simulink model "MMMS_v1_dynamics"  (R2024a)
settings: Solver=VariableStepAuto  StartTime=0.0  StopTime=120  FixedStep=0.001  RelTol=1e-3
InitFcn:
  | %rho_0t=[0.29;0.29;0.29]; %m
  | %V_0t=[-0.001;-0.001;0];%[-0.0005;-0.0005;0];
  | %w_t=[0;0;-0.002];
  | 
  | 
  | %rho_0t=[0.3;0.3;0.2]; %m
  | %V_0t=[-0.001;-0.001;0];%[-0.0005;-0.0005;0];
  | %w_t=[0;0;-0.001];
values from neighbouring files (symbols this model uses):
  Dt = 0.1    [main_EKF.m]
  g_cm = zeros(4,4,n)    [Initiate_KUKA_inv.m]    (also in Main_MMMS.m; test_KUKA_elements.m)
  g_It00 = [eye(3) rho_It;0 0 0 1]    [main_EKF.m]
  iota0 = eye(6,6)    [Initiate_KUKA_inv.m]    (also in Main_MMMS.m; test_KUKA_elements.m)
  K_d = 10*[1.3*eye(3) zeros(3);zeros(3) 0.8*eye(3)]    [Initiate_FQ.m]    (also in Initiate_KUKA_inv.m = 5*[0.7*eye(3) zeros(3);zeros(3) 0.5*eye(3)]; MMMS_Initiate_FQ.m; Main_MMMS.m = 5*[0.7*eye(3) zeros(3);zeros(3) 0.5*eye(3)]; test_KUKA_elements.m = 50*[0.7*eye(3) zeros(3);zeros(3) 0.5*eye(3)])
  K_i = 5*[0.1*eye(3) zeros(3);zeros(3) 0.01*eye(3)]    [Initiate_FQ.m]    (also in Initiate_KUKA_inv.m = 5*[0.01*eye(3) zeros(3);zeros(3) 0.001*eye(3)]; MMMS_Initiate_FQ.m; Main_MMMS.m = 5*[0.01*eye(3) zeros(3);zeros(3) 0.001*eye(3)]; test_KUKA_elements.m = 50*[0.01*eye(3) zeros(3);zeros(3) 0.001*eye(3)])
  K_p = 100*[0.1 0 0 0 0 0;0 0.1 0 0 0 0; 0 0 0.1 0 0 0; 0 0 0 0.01 0 0 ... (first row only)    [Initiate_FQ.m]    (also in Initiate_KUKA_inv.m = 5*[0.1 0 0 0 0 0;0 0.1 0 0 0 0; 0 0 0.1 0 0 0; 0 0 0 0.01 0 ; MMMS_Initiate_FQ.m; Main_MMMS.m = 5*[0.1 0 0 0 0 0;0 0.1 0 0 0 0; 0 0 0.1 0 0 0; 0 0 0 0.01 0 ; test_KUKA_elements.m = 50*[0.1 0 0 0 0 0;0 0.1 0 0 0 0; 0 0 0.1 0 0 0; 0 0 0 0.01 0)
  K_w = 200*eye(7)    [Initiate_FQ.m]    (also in MMMS_Initiate_FQ.m)
  K_wd = 2*eye(7)    [Initiate_FQ.m]    (also in MMMS_Initiate_FQ.m)
  m = randn(s,total_time_steps,6)*chol(R)    [main_EKF.m]
  M0 = M_temp.M0.data(:,:,1)    [Initiate_FQ.m]    (also in MMMS_Initiate_FQ.m; test_KUKA_elements.m)
  m0 = robot.Bodies{1,n+1}.Mass    [Initiate_KUKA_inv.m]    (also in Main_MMMS.m; test_KUKA_elements.m)
  m0_frak = diag_M(1:6,1:6)    [Initiate_KUKA_inv.m]    (also in Main_MMMS.m; make_uncertain.m = diag_M_unc(1:6,1:6); test_KUKA_elements.m)
  M0m = M_temp.M0m.data(:,:,1)    [Initiate_FQ.m]    (also in MMMS_Initiate_FQ.m; test_KUKA_elements.m)
  m_diag = diag_M(7:end,7:end)    [Initiate_KUKA_inv.m]    (also in Main_MMMS.m; make_uncertain.m = diag_M_unc(7:end,7:end); test_KUKA_elements.m)
  M_t = (((Adjoint(g_It))'\M_t_body)/(Adjoint(g_It)))    [Initiate_FQ.m]    (also in Initiate_KUKA_inv.m = [eye(3)*mt zeros(3); zeros(3) eye(3)*80]; MMMS_Initiate_FQ.m; Main_MMMS.m = [eye(3)*mt zeros(3); zeros(3) eye(3)*80]; test_KUKA_elements.m = [eye(3)*mt zeros(3); zeros(3) eye(3)*80])
  M_t_body = [eye(3)*mt zeros(3); zeros(3) eye(3)*0.416667]    [Initiate_FQ.m]    (also in MMMS_Initiate_FQ.m)
  mm = zeros(1,n)    [Initiate_KUKA_inv.m]    (also in Main_MMMS.m; test_KUKA_elements.m)
  mu = P0    [Initiate_FQ.m]    (also in Initiate_KUKA_inv.m = zeros(6,1); MMMS_Initiate_FQ.m; Main_MMMS.m = zeros(6,1); make_uncertain.m = P0_unc)
  mu_t = inv((Adjoint(g_It))')*M_t_body*[V_It;w_t]    [Initiate_FQ.m]    (also in Initiate_KUKA_inv.m = M_t*[V_0t;w_t]; MMMS_Initiate_FQ.m; Main_MMMS.m = M_t*[V_0t;w_t]; make_uncertain.m = inv((Adjoint(g_It))')*M_t_body_unc*[V_It;w_t])
  noise_st = 0.000005    (= 5e-06)    [main_EKF.m]
  q_dot_m = [0;0;0;0;0;0;0]    [Initiate_FQ.m]    (also in Initiate_KUKA_inv.m; MMMS_Initiate_FQ.m; Main_MMMS.m; test_KUKA_elements.m = [0])
  q_m = [0.2;1.2;0.3;2.5;0.5;1.5;0.6]    [Initiate_FQ.m]    (also in Initiate_KUKA_inv.m = [0;0;0;0;0;0;0]; MMMS_Initiate_FQ.m = [0.2;0.2;0.3;0.5;0.5;0.5;0.6]; Main_MMMS.m = [0;0;0;0;0;0;0]; test_KUKA_elements.m = [0.2;1.2;0.3;1.8;0.5;1.3;0.6])
  rho_It = [-0.3;-0.3;-0.1]    [Initiate_FQ.m]    (also in MMMS_Initiate_FQ.m = [0;0;1.7])
  s = RandStream.create('mrg32k3a','NumStreams',1)    [main_EKF.m]
  sc_size = 1    [Initiate_KUKA_inv.m]    (also in Main_MMMS.m; test_KUKA_elements.m)
  V_It = [0.01;0.01;0]    [Initiate_FQ.m]    (also in MMMS_Initiate_FQ.m = [0.001;0.001;0])
  Xi_m_matrix = zeros(6*n,n)    [Initiate_KUKA_inv.m]    (also in Main_MMMS.m)
undefined symbols (not defined in the file or in its folder): g_cm0, I0, Im, Mm, X, Xi_m, Y, Z
libraries: nesl_utility x314, sm_lib x231, robotcorelib x30, simulink x12
(part 1 of 13)
settings Model: Creator=Bmmog  LastModifiedBy=Bmmog
settings SolverCC: ZeroCrossAlgorithm=Adaptive
settings DataIOCC: ReturnWorkspaceOutputsName=tp1ae71780_9f9b_41fc_80d6_93119145c185
settings DebuggingCC: UnconnectedInputMsg=warning  UnconnectedOutputMsg=warning  UnconnectedLineMsg=warning
settings ModelReferenceCC: EnableRefExpFcnMdlSchedulingChecks=on
settings RTWCC: GPUComputeCapability=3.5  DLArmComputeVersion=19.05
settings ExplorerConfigSet: InternalSimMechanicsExplorerSettings="<ExplorerConfiguration><canonicalview>default</canonicalview><AnimationSetting><BasePlaybackSpeed>1.0</BasePlaybackSpeed><PlaybackSpeedFactor>8.0</PlaybackSpeedFactor></AnimationSetting><TilePanel><TileInfo><Tiles Columns=\"1\" Count=\"1\" Rows=\"1\"><Column Weight=\"1\"/><Row Weight=\"1\"/><Tile Height=\"1\" Width=\"1\" X=\"0\" Y=\"0\"/></Tiles></TileInfo><SceneInfo><SceneViewer><BGColor><R>1</R><G>1</G><B>1</B></BGColor><Camera><DoPerspective>off</DoPerspective><Position><X>14.9326991217614395</X><Y>-1.09548928723552041</Y><Z>10.2239075521242828</Z></Position><Center><X>11.9633929326695281</X><Y>-0.827691225044008383</Y><Z>8.31444606315609391</Z></Center><Up><X>-0.521882593040954079</X><Y>0.171482170510200094</Y><Z>0.835603030318799456</Z></Up><ViewLimDist>1</ViewLimDist><YLim>2.32554507561611068</YLim><XLim>3.37013417515515057</XLim></Camera></SceneViewer></SceneInfo></TilePanel><MechEditorPanel><Cameras/><GfxPanelCameraMap/><VideoCreator><PlaybackSpeedRatio>1.0</PlaybackSpeedRatio><FrameRate>30</FrameRate><VideoFormat>Motion JPEG AVI</VideoFormat><FrameSize>auto</FrameSize></VideoCreator></MechEditorPanel></ExplorerConfiguration>"

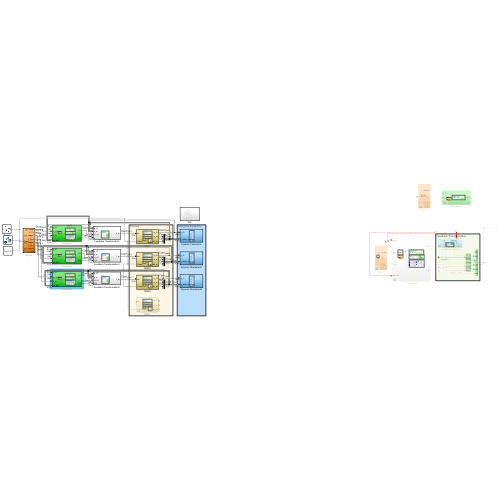
[thumbnail: Simulink's stored preview of the top-level diagram]
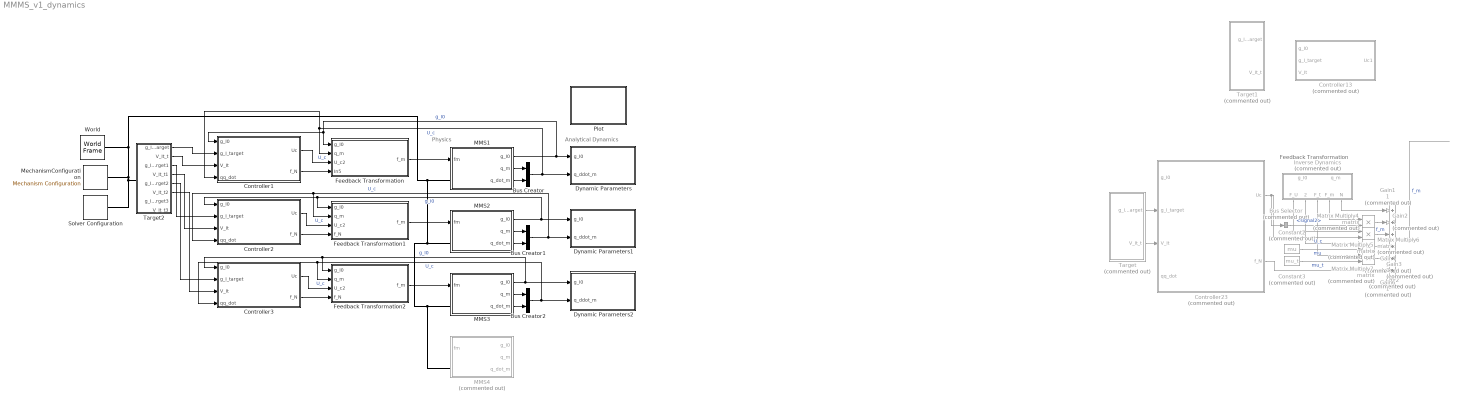
== system MMMS_v1_dynamics ==
  note: Analytical Dynamics
  note: Physics
  note: Feedback Transformation
  Add2 : Sum  Commented=on  Inputs=++++++
  Bus Creator : BusCreator  Inputs=2
  Bus Creator1 : BusCreator  Inputs=2
  Bus Creator2 : BusCreator  Inputs=2
  Bus Selector : BusSelector  Commented=on  OutputSignals=signal2
  Constant2 : Constant  Commented=on  Value=mu
  Constant3 : Constant  Commented=on  Value=mu_t
  Controller1 : Subsystem
  Controller13 : Subsystem  Commented=on
  Controller2 : Subsystem
  Controller23 : Subsystem  Commented=on
  Controller3 : Subsystem
  Dynamic Parameters : Subsystem
  Dynamic Parameters1 : Subsystem
  Dynamic Parameters2 : Subsystem
  Feedback Transformation : Subsystem
  Feedback Transformation1 : Subsystem
  Feedback Transformation2 : Subsystem
  Gain{1..4,6} (5 alike) : Gain  Commented=on
  Inverse Dynamics : Subsystem  Commented=on
  MMS1 : Subsystem
  MMS2 : Subsystem
  MMS3 : Subsystem
  MMS4 : Subsystem  Commented=on
  Matrix Multiply{4..7} (4 alike) : Product  Commented=on  Multiplication=Matrix(*)
  MechanismConfiguration : sm_lib/Utilities/Mechanism Configuration  UniformGravity=Constant  GravityVector=[0 0 0]  GravityVectorUnits=m/s^2  LinearizationDelta=0.001  JointModeTransitionNonlinearIterations=2
  Plot : Subsystem
  Solver Configuration : nesl_utility/Solver Configuration  PhysicalDomain=network_engine_domain  SubClassName=solver  LeftPortType=input  RightPortType=generic  Tones=[]  Harmonics=[]  SimulateNoise=off  Profile=off  UseLocalSampling=off  EnableSwitchedLinearOptims=on  FrequencyDomain=off  UseCCode=off  RelTol=0.001  AbsTol=0.001  MinStep=1e-09  ToWorkspace=off  RevertToSquareIcSolve=off  NumHomotopyIterations=100  PhasorMode=off  PhasorModeNumHarmonics=1  ConsistencySolver=NEWTON_FTOL  IndexReductionMethod=DerivativeReplacement  DoDC=off  ResidualTolerance=1e-9  ConsistencyTolSource=GLOBAL  ConsistencyAbsTol=0.001  ConsistencyRelTol=0.001  ConsistencyTolFactor=0.001  UseLocalSolver=off  LocalSolverChoice=NE_BACKWARD_EULER_ADVANCER  ResolveIndetEquations=on  FunctionEvalNumThread=1  LocalSolverSampleTime=0.001  DoFixedCost=off  MaxNonlinIter=3  MaxModeIter=2  ComputeImpulses=off  ImpulseIterations=2  LinearAlgebra=Full  LinearAlgebraNumThread=0  EquationFormulation=NE_TIME_EF  DelaysMemoryBudget=1024  AutomaticFiltering=off  FilteringTimeConstant=0.001  PartitionStorageMethod=AS_NEEDED  PartitionMemoryBudget=1024  PartitionMethod=ROBUST  MultibodyUseLocalSolver=off  MultibodyLocalSolverChoice=ODE1  MultibodyLocalSolverSampleTime=0.001
  Target : Subsystem  Commented=on
  Target1 : Subsystem  Commented=on
  Target2 : Subsystem
  World : sm_lib/Frames and Transforms/World Frame
  wires:
  MMS1/2(q_m) -> Bus Creator/1
  MMS1/3(q_dot_m) -> Bus Creator/2
  Gain3/1 -> Add2/5
  Constant3/1 -> Matrix Multiply7/2  "mu_t"
  Controller23/2(f_N) -> Gain6/1
  Gain4/1 -> Add2/4
  Inverse Dynamics/1(F_U) -> Matrix Multiply5/1
  Inverse Dynamics/5(N) -> Gain1/1
  Gain6/1 -> Add2/6
  Matrix Multiply6/1 -> Gain4/1
  Matrix Multiply7/1 -> Gain3/1
  Gain2/1 -> Add2/2
  Inverse Dynamics/2(F_mu) -> Matrix Multiply6/1
  Target/1(g_I_target) -> Controller23/2(g_I_target)
  Inverse Dynamics/4(F_m) -> Matrix Multiply4/1
  Add2/1 -> ?  "f_m"
  Gain1/1 -> Add2/1
  Constant2/1 -> Matrix Multiply6/2  "mu"
  Controller23/1(Uc) -> Matrix Multiply5/2, Bus Selector/1  "U_c"
  Inverse Dynamics/3(F_t) -> Matrix Multiply7/1
  Matrix Multiply5/1 -> Add2/3  "f_m"
  ? -> Controller23/4(qq_dot)
  Matrix Multiply4/1 -> Gain2/1
  ? -> Inverse Dynamics/2("q_m ")
  ? -> Controller23/1(g_I0)  "g_I0"
  Target/2(V_It_t) -> Controller23/3(V_It)
  Bus Selector/1 -> Matrix Multiply4/2  "<signal2>"
  Bus Creator/1 -> Feedback Transformation/2(q_m), Controller1/4(qq_dot), Dynamic Parameters/2(q_ddot_m)  "U_c"
  Target2/1(g_I_target) -> Controller1/2(g_I_target)
  Target2/2(V_It_t) -> Controller1/3(V_It)
  MMS1/1(g_I0) -> Controller1/1(g_I0), Feedback Transformation/1(g_I0), Dynamic Parameters/1(g_I0)  "g_I0"
  Controller1/1(Uc) -> Feedback Transformation/3(U_c2)  "U_c"
  Controller1/2(f_N) -> Feedback Transformation/4(In5)
  Feedback Transformation/1(f_m) -> MMS1/1(fm)
  MMS2/2(q_m) -> Bus Creator1/1
  MMS2/3(q_dot_m) -> Bus Creator1/2
  MMS2/1(g_I0) -> Feedback Transformation1/1(g_I0), Controller2/1(g_I0), Dynamic Parameters1/1(g_I0)  "g_I0"
  Bus Creator1/1 -> Feedback Transformation1/2(q_m), Controller2/4(qq_dot), Dynamic Parameters1/2(q_ddot_m)  "U_c"
  Controller2/1(Uc) -> Feedback Transformation1/3(U_c2)  "U_c"
  Controller2/2(f_N) -> Feedback Transformation1/4(f_N)
  Target2/3(g_I_target1) -> Controller2/2(g_I_target)
  Target2/4(V_It_t1) -> Controller2/3(V_It)
  Feedback Transformation1/1(f_m) -> MMS2/1(fm)
  MMS3/1(g_I0) -> Feedback Transformation2/1(g_I0), Controller3/1(g_I0), Dynamic Parameters2/1(g_I0)  "g_I0"
  MMS3/2(q_m) -> Bus Creator2/1
  MMS3/3(q_dot_m) -> Bus Creator2/2
  Bus Creator2/1 -> Feedback Transformation2/2(q_m), Controller3/4(qq_dot), Dynamic Parameters2/2(q_ddot_m)  "U_c"
  Controller3/2(f_N) -> Feedback Transformation2/4(f_N)
  Controller3/1(Uc) -> Feedback Transformation2/3(U_c2)  "U_c"
  Target2/5(g_I_target2) -> Controller3/2(g_I_target)
  Target2/6(V_It_t2) -> Controller3/3(V_It)
  Feedback Transformation2/1(f_m) -> MMS3/1(fm)
  connections:
  MechanismConfiguration/RConn1 -- Target2/LConn1 -- Solver Configuration/RConn1 -- MMS4/LConn1 -- MMS3/LConn1 -- MMS2/LConn1 -- MMS1/LConn1 -- World/RConn1

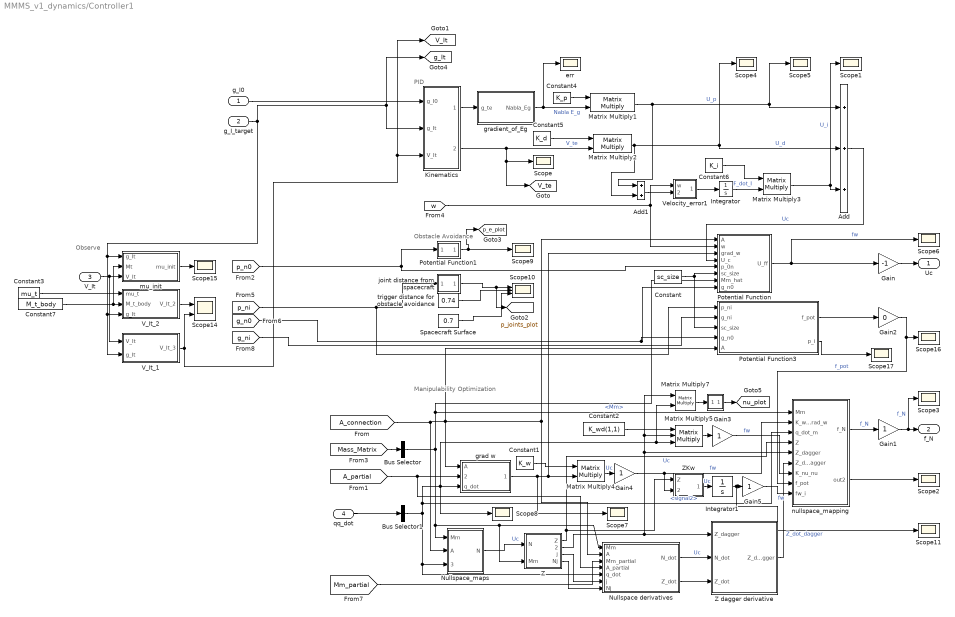
== system MMMS_v1_dynamics/Controller1 ==
  note: PID
  note: Manipulability Optimization
  note: Obstacle Avoidance
  note: Observe
  g_I0 : Inport
  g_I_target : Inport  Port=2
  V_It : Inport  Port=3
  qq_dot : Inport  Port=4
  " " : MATLAB Function  TreatAsAtomicUnit=on
  Add : Sum  Inputs=+++
  Add1 : Sum
  Bus Selector : BusSelector  OutputSignals=Mm
  Bus Selector1 : BusSelector  OutputSignals=signal2
  Constant : Constant  Value=sc_size
  Constant1 : Constant  Value=K_w
  Constant2 : Constant  Value=K_wd(1,1)
  Constant3 : Constant  Value=mu_t
  Constant4 : Constant  Value=K_p
  Constant5 : Constant  Value=K_d
  Constant6 : Constant  Value=K_i
  Constant7 : Constant  Value=M_t_body
  Gain : Gain  Gain=-1
  Gain{1,3..5} (4 alike) : Gain
  Gain2 : Gain  Gain=0
  Integrator : Integrator
  Integrator1 : Integrator
  Kinematics : Subsystem
  Matrix Multiply{1..4,7} (5 alike) : Product  Multiplication=Matrix(*)
  Matrix Multiply5 : Product  Inputs=3  Multiplication=Matrix(*)
  Nullspace derivatives : MATLAB Function  TreatAsAtomicUnit=on
  Nullspace_maps : MATLAB Function  TreatAsAtomicUnit=on
  Potential Function : MATLAB Function  TreatAsAtomicUnit=on
  Potential Function1 : MATLAB Function  TreatAsAtomicUnit=on
  Potential Function3 : MATLAB Function  TreatAsAtomicUnit=on
  Scope{,1..9,11,15..17} (14 alike) : Scope
  Scope10 : Scope  NumInputPorts=3
  Scope14 : Scope  NumInputPorts=2
  Spacecraft Surface : Constant  Value=0.7
  V_It_1 : MATLAB Function  TreatAsAtomicUnit=on
  V_It_2 : MATLAB Function  TreatAsAtomicUnit=on
  Velocity_error1 : MATLAB Function  TreatAsAtomicUnit=on
  Z : MATLAB Function  TreatAsAtomicUnit=on
  Z dagger derivative : MATLAB Function  TreatAsAtomicUnit=on
  ZKw : MATLAB Function  TreatAsAtomicUnit=on
  err : Scope
  grad w : MATLAB Function  TreatAsAtomicUnit=on
  gradient_of_Eg : MATLAB Function  TreatAsAtomicUnit=on
  joint distance from spacecraft : MATLAB Function  TreatAsAtomicUnit=on
  mu_init : MATLAB Function  TreatAsAtomicUnit=on
  nullspace_mapping : MATLAB Function  TreatAsAtomicUnit=on
  trigger distance for obstacle avoidance : Constant  Value=0.74
  Uc : Outport
  f_N : Outport  Port=2
  tag scope: V_It=global, V_te=global, g_It=global, nu_plot=global, p_e_plot=global, p_joints_plot=global
  wires:
  [A_connection] -> Potential Function3/5(A), Potential Function/1(A), Nullspace derivatives/2(A), grad w/1(A), Nullspace_maps/2(A)
  [A_partial] -> grad w/2(A_partial), Nullspace derivatives/4(A_partial)
  qq_dot/1 -> Bus Selector1/1
  [Mass_Matrix] -> Bus Selector/1
  Bus Selector/1 -> Nullspace_maps/1(Mm), Z/2(Mm), Nullspace derivatives/1(Mm), Potential Function/7(Mm_hat), nullspace_mapping/1(Mm)  "<Mm>"
  Gain/1 -> Uc/1
  g_I0/1 -> Kinematics/1(g_I0)
  Add/1 -> Potential Function/4(U_c)  "Uc"
  Kinematics/1(g_te1) -> gradient_of_Eg/1(g_te)
  Add1/1 -> Velocity_error1/2(in)
  Matrix Multiply2/1 -> Scope4/1, Add/2, Add1/2  "U_d"
  gradient_of_Eg/1(Nabla_Eg) -> err/1, Matrix Multiply1/2  "Nabla E_g"
  Constant4/1 -> Matrix Multiply1/1
  Kinematics/2(V_te) -> [V_te], Scope/1, Matrix Multiply2/2  "V_te"
  Constant6/1 -> Matrix Multiply3/1
  Integrator/1 -> Matrix Multiply3/2  "F_dot_I"
  Matrix Multiply1/1 -> Scope5/1, Add/1, Add1/1  "U_p"
  Constant5/1 -> Matrix Multiply2/1
  Bus Selector1/1 -> nullspace_mapping/3(q_dot_m), Scope8/1, grad w/3(q_dot), Matrix Multiply7/2, Matrix Multiply5/3, Nullspace derivatives/5(q_dot), Nullspace_maps/3(q_dot_m)  "<signal2>"
  Gain1/1 -> f_N/1, Scope3/1  "f_N"
  Constant1/1 -> Matrix Multiply4/1
  grad w/1(grad_w) -> Scope7/1, Potential Function/3(grad_w), Matrix Multiply4/2
  Matrix Multiply5/1 -> Gain3/1
  Constant2/1 -> Matrix Multiply5/1
  Matrix Multiply4/1 -> Gain4/1  "Uc"
  Matrix Multiply3/1 -> Scope1/1, Add/3  "U_i"
  nullspace_mapping/1(f_N) -> Gain1/1  "f_N"
  [w] -> Potential Function/2(w), Velocity_error1/1(w)
  Potential Function/1(U_ff) -> Gain/1, Scope6/1  "fw"
  Velocity_error1/1(out) -> Integrator/1
  [p_n0] -> Potential Function1/1(p_0n), Potential Function/5(p_0n)
  Potential Function1/1(w_p) -> Scope9/1, [p_e_plot]
  [p_ni] -> joint distance from spacecraft/1(p_joints), Potential Function3/1(p_ni)
  joint distance from spacecraft/1(pnorm) -> [p_joints_plot], Scope10/1
  [g_n0] -> Potential Function3/4(g_n0), Potential Function/8(g_n0)
  Potential Function3/1(f_pot) -> Gain2/1
  Constant/1 -> Potential Function3/3(sc_size), Potential Function/6(sc_size)
  trigger distance for obstacle avoidance/1 -> Scope10/2
  Gain3/1 -> nullspace_mapping/7(K_nu_nu)  "fw"
  Nullspace derivatives/1(N_dot) -> Z dagger derivative/2(N_dot)  "Uc"
  Nullspace derivatives/2(Z_dot) -> Z dagger derivative/3(Z_dot)
  Z dagger derivative/1(Z_dot_dagger) -> nullspace_mapping/6(Z_dot_dagger)  "Z_dot_dagger"
  Nullspace_maps/1(N) -> Z/1(N)  "Uc"
  [Mm_partial] -> Nullspace derivatives/3(Mm_partial)
  Z/1(Z) -> ZKw/1(Z), nullspace_mapping/4(Z)  "Uc"
  Gain4/1 -> ZKw/2(K_w_grad_w), nullspace_mapping/2(K_w_grad_w)  "fw"
  nullspace_mapping/2(out2) -> Scope2/1
  Z/2(Z_dagger) -> Z dagger derivative/1(Z_dagger), nullspace_mapping/5(Z_dagger), Matrix Multiply7/1, Matrix Multiply5/2
  ZKw/1(out) -> Integrator1/1  "Uc"
  Integrator1/1 -> Scope11/1, Gain5/1
  Gain5/1 -> nullspace_mapping/9(fw_i)  "fw"
  V_It/1 -> V_It_1/1(V_It), mu_init/3(V_It)
  Constant3/1 -> V_It_2/1(mu_t)
  mu_init/1(mu_init) -> Scope15/1
  Constant7/1 -> mu_init/2(Mt), V_It_2/2(M_t_body)
  Gain2/1 -> Scope16/1, nullspace_mapping/8(f_pot)  "f_pot"
  Z/3(j) -> Nullspace derivatives/6(j)
  Z/4(Nj) -> Nullspace derivatives/7(Nj)
  V_It_2/1(V_It_2) -> Scope14/1
  V_It_1/1(V_It_3) -> Scope14/2, Kinematics/3(V_It), [V_It]
  Spacecraft Surface/1 -> Scope10/3
  [g_ni] -> Potential Function3/2(g_ni)
  Potential Function3/2(p_i) -> Scope17/1
  g_I_target/1 -> Kinematics/2(g_It), [g_It], V_It_1/2(g_It), V_It_2/3(g_It), mu_init/1(g_It)
  " "/1(normA) -> [nu_plot]
  Matrix Multiply7/1 -> " "/1(A)

== system MMMS_v1_dynamics/Controller13 ==
  note: PID
  note: Observe
  g_I0 : Inport
  g_I_target : Inport  Port=2
  V_It : Inport  Port=3
  Add : Sum  Inputs=+++
  Add1 : Sum
  Constant3 : Constant  Value=mu_t
  Constant4 : Constant  Value=K_p
  Constant5 : Constant  Value=K_d
  Constant6 : Constant  Value=K_i
  Constant7 : Constant  Value=M_t_body
  From4 : From  Commented=on  GotoTag=w
  Gain1 : Gain  Gain=-1
  Integrator : Integrator
  Kinematics : Subsystem
  Matrix Multiply1 : Product  Multiplication=Matrix(*)
  Matrix Multiply2 : Product  Multiplication=Matrix(*)
  Matrix Multiply3 : Product  Multiplication=Matrix(*)
  Scope : Scope
  Scope1 : Scope  NumInputPorts=3
  Scope14 : Scope  NumInputPorts=2
  Scope15 : Scope
  V_It_1 : MATLAB Function  TreatAsAtomicUnit=on
  V_It_2 : MATLAB Function  TreatAsAtomicUnit=on
  Velocity_error1 : MATLAB Function  Commented=on  TreatAsAtomicUnit=on
  err : Scope
  gradient_of_Eg : MATLAB Function  TreatAsAtomicUnit=on
  mu_init : MATLAB Function  TreatAsAtomicUnit=on
  Uc1 : Outport
  tag scope: V_It=global, V_te=global, g_It=global
  wires:
  g_I0/1 -> Kinematics/1(g_I0)
  Kinematics/1(g_te1) -> gradient_of_Eg/1(g_te)
  Matrix Multiply2/1 -> Add/2, Scope1/2, Add1/2  "U_d"
  gradient_of_Eg/1(Nabla_Eg) -> err/1, Matrix Multiply1/2  "Nabla E_g"
  Constant4/1 -> Matrix Multiply1/1
  Kinematics/2(V_te) -> [V_te], Scope/1, Matrix Multiply2/2  "V_te"
  Constant6/1 -> Matrix Multiply3/1
  Integrator/1 -> Matrix Multiply3/2  "F_dot_I"
  Matrix Multiply1/1 -> Scope1/1, Add/1, Add1/1  "U_p"
  Constant5/1 -> Matrix Multiply2/1
  Matrix Multiply3/1 -> Add/3, Scope1/3  "U_i"
  From4/1 -> Velocity_error1/1(w)
  Add1/1 -> Integrator/1
  V_It/1 -> V_It_1/1(V_It), mu_init/3(V_It)
  Constant3/1 -> V_It_2/1(mu_t)
  mu_init/1(mu_init) -> Scope15/1
  Constant7/1 -> mu_init/2(Mt), V_It_2/2(M_t_body)
  V_It_2/1(V_It_2) -> Scope14/1
  V_It_1/1(V_It_3) -> Scope14/2, Kinematics/3(V_It), [V_It]
  g_I_target/1 -> [g_It], Kinematics/2(g_It), V_It_1/2(g_It), V_It_2/3(g_It), mu_init/1(g_It)
  Add/1 -> Gain1/1  "Uc"
  Gain1/1 -> Uc1/1

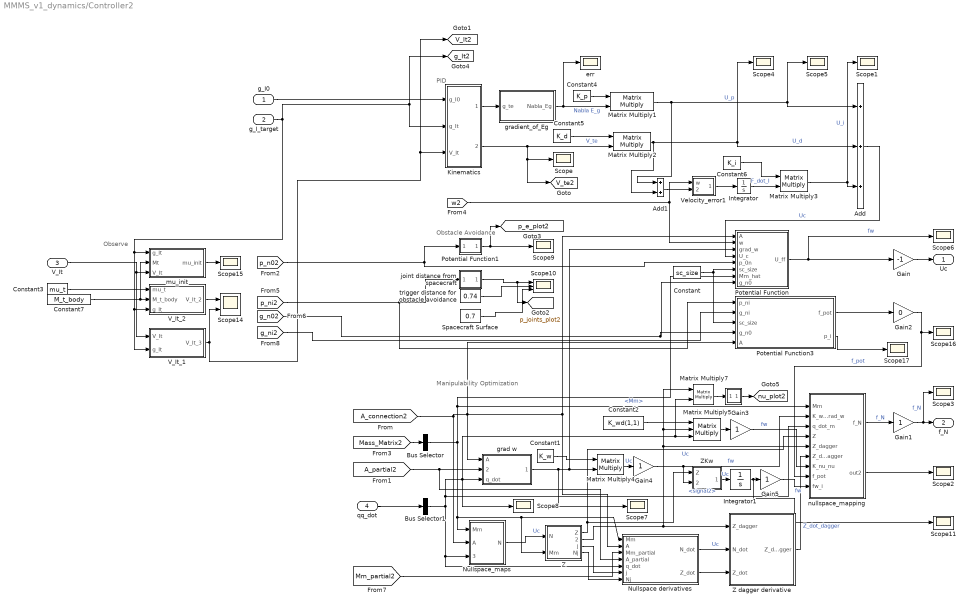
== system MMMS_v1_dynamics/Controller2 ==
  note: Observe
  note: Obstacle Avoidance
  note: Manipulability Optimization
  note: PID
  g_I0 : Inport
  g_I_target : Inport  Port=2
  V_It : Inport  Port=3
  qq_dot : Inport  Port=4
  " " : MATLAB Function  TreatAsAtomicUnit=on
  Add : Sum  Inputs=+++
  Add1 : Sum
  Bus Selector : BusSelector  OutputSignals=Mm
  Bus Selector1 : BusSelector  OutputSignals=signal2
  Constant : Constant  Value=sc_size
  Constant1 : Constant  Value=K_w
  Constant2 : Constant  Value=K_wd(1,1)
  Constant3 : Constant  Value=mu_t
  Constant4 : Constant  Value=K_p
  Constant5 : Constant  Value=K_d
  Constant6 : Constant  Value=K_i
  Constant7 : Constant  Value=M_t_body
  Gain : Gain  Gain=-1
  Gain{1,3..5} (4 alike) : Gain
  Gain2 : Gain  Gain=0
  Integrator : Integrator
  Integrator1 : Integrator
  Kinematics : Subsystem
  Matrix Multiply{1..4,7} (5 alike) : Product  Multiplication=Matrix(*)
  Matrix Multiply5 : Product  Inputs=3  Multiplication=Matrix(*)
  Nullspace derivatives : MATLAB Function  TreatAsAtomicUnit=on
  Nullspace_maps : MATLAB Function  TreatAsAtomicUnit=on
  Potential Function : MATLAB Function  TreatAsAtomicUnit=on
  Potential Function1 : MATLAB Function  TreatAsAtomicUnit=on
  Potential Function3 : MATLAB Function  TreatAsAtomicUnit=on
  Scope{,1..9,11,15..17} (14 alike) : Scope
  Scope10 : Scope  NumInputPorts=3
  Scope14 : Scope  NumInputPorts=2
  Spacecraft Surface : Constant  Value=0.7
  V_It_1 : MATLAB Function  TreatAsAtomicUnit=on
  V_It_2 : MATLAB Function  TreatAsAtomicUnit=on
  Velocity_error1 : MATLAB Function  TreatAsAtomicUnit=on
  Z : MATLAB Function  TreatAsAtomicUnit=on
  Z dagger derivative : MATLAB Function  TreatAsAtomicUnit=on
  ZKw : MATLAB Function  TreatAsAtomicUnit=on
  err : Scope
  grad w : MATLAB Function  TreatAsAtomicUnit=on
  gradient_of_Eg : MATLAB Function  TreatAsAtomicUnit=on
  joint distance from spacecraft : MATLAB Function  TreatAsAtomicUnit=on
  mu_init : MATLAB Function  TreatAsAtomicUnit=on
  nullspace_mapping : MATLAB Function  TreatAsAtomicUnit=on
  trigger distance for obstacle avoidance : Constant  Value=0.74
  Uc : Outport
  f_N : Outport  Port=2
  tag scope: V_It2=global, V_te2=global, g_It2=global, nu_plot2=global, p_e_plot2=global, p_joints_plot2=global
  wires:
  Matrix Multiply7/1 -> " "/1(A)
  " "/1(normA) -> [nu_plot2]
  g_I_target/1 -> mu_init/1(g_It), V_It_2/3(g_It), V_It_1/2(g_It), [g_It2], Kinematics/2(g_It)
  Potential Function3/2(p_i) -> Scope17/1
  [g_ni2] -> Potential Function3/2(g_ni)
  Spacecraft Surface/1 -> Scope10/3
  V_It_1/1(V_It_3) -> [V_It2], Kinematics/3(V_It), Scope14/2
  V_It_2/1(V_It_2) -> Scope14/1
  Z/4(Nj) -> Nullspace derivatives/7(Nj)
  Z/3(j) -> Nullspace derivatives/6(j)
  Gain2/1 -> nullspace_mapping/8(f_pot), Scope16/1  "f_pot"
  Constant7/1 -> V_It_2/2(M_t_body), mu_init/2(Mt)
  mu_init/1(mu_init) -> Scope15/1
  Constant3/1 -> V_It_2/1(mu_t)
  V_It/1 -> mu_init/3(V_It), V_It_1/1(V_It)
  Gain5/1 -> nullspace_mapping/9(fw_i)  "fw"
  Integrator1/1 -> Gain5/1, Scope11/1
  ZKw/1(out) -> Integrator1/1  "Uc"
  Z/2(Z_dagger) -> Matrix Multiply5/2, Matrix Multiply7/1, nullspace_mapping/5(Z_dagger), Z dagger derivative/1(Z_dagger)
  nullspace_mapping/2(out2) -> Scope2/1
  Gain4/1 -> nullspace_mapping/2(K_w_grad_w), ZKw/2(K_w_grad_w)  "fw"
  Z/1(Z) -> nullspace_mapping/4(Z), ZKw/1(Z)  "Uc"
  [Mm_partial2] -> Nullspace derivatives/3(Mm_partial)
  Nullspace_maps/1(N) -> Z/1(N)  "Uc"
  Z dagger derivative/1(Z_dot_dagger) -> nullspace_mapping/6(Z_dot_dagger)  "Z_dot_dagger"
  Nullspace derivatives/2(Z_dot) -> Z dagger derivative/3(Z_dot)
  Nullspace derivatives/1(N_dot) -> Z dagger derivative/2(N_dot)  "Uc"
  Gain3/1 -> nullspace_mapping/7(K_nu_nu)  "fw"
  trigger distance for obstacle avoidance/1 -> Scope10/2
  Constant/1 -> Potential Function/6(sc_size), Potential Function3/3(sc_size)
  Potential Function3/1(f_pot) -> Gain2/1
  [g_n02] -> Potential Function/8(g_n0), Potential Function3/4(g_n0)
  joint distance from spacecraft/1(pnorm) -> Scope10/1, [p_joints_plot2]
  [p_ni2] -> Potential Function3/1(p_ni), joint distance from spacecraft/1(p_joints)
  Potential Function1/1(w_p) -> [p_e_plot2], Scope9/1
  [p_n02] -> Potential Function/5(p_0n), Potential Function1/1(p_0n)
  Velocity_error1/1(out) -> Integrator/1
  Potential Function/1(U_ff) -> Scope6/1, Gain/1  "fw"
  [w2] -> Velocity_error1/1(w), Potential Function/2(w)
  nullspace_mapping/1(f_N) -> Gain1/1  "f_N"
  Matrix Multiply3/1 -> Add/3, Scope1/1  "U_i"
  Matrix Multiply4/1 -> Gain4/1  "Uc"
  Constant2/1 -> Matrix Multiply5/1
  Matrix Multiply5/1 -> Gain3/1
  grad w/1(grad_w) -> Matrix Multiply4/2, Potential Function/3(grad_w), Scope7/1
  Constant1/1 -> Matrix Multiply4/1
  Gain1/1 -> Scope3/1, f_N/1  "f_N"
  Bus Selector1/1 -> Nullspace_maps/3(q_dot_m), Nullspace derivatives/5(q_dot), Matrix Multiply5/3, Matrix Multiply7/2, grad w/3(q_dot), Scope8/1, nullspace_mapping/3(q_dot_m)  "<signal2>"
  Constant5/1 -> Matrix Multiply2/1
  Matrix Multiply1/1 -> Add1/1, Add/1, Scope5/1  "U_p"
  Integrator/1 -> Matrix Multiply3/2  "F_dot_I"
  Constant6/1 -> Matrix Multiply3/1
  Kinematics/2(V_te) -> Matrix Multiply2/2, Scope/1, [V_te2]  "V_te"
  Constant4/1 -> Matrix Multiply1/1
  gradient_of_Eg/1(Nabla_Eg) -> Matrix Multiply1/2, err/1  "Nabla E_g"
  Matrix Multiply2/1 -> Add1/2, Add/2, Scope4/1  "U_d"
  Add1/1 -> Velocity_error1/2(in)
  Kinematics/1(g_te1) -> gradient_of_Eg/1(g_te)
  Add/1 -> Potential Function/4(U_c)  "Uc"
  g_I0/1 -> Kinematics/1(g_I0)
  Gain/1 -> Uc/1
  Bus Selector/1 -> nullspace_mapping/1(Mm), Potential Function/7(Mm_hat), Nullspace derivatives/1(Mm), Z/2(Mm), Nullspace_maps/1(Mm)  "<Mm>"
  [Mass_Matrix2] -> Bus Selector/1
  qq_dot/1 -> Bus Selector1/1
  [A_partial2] -> Nullspace derivatives/4(A_partial), grad w/2(A_partial)
  [A_connection2] -> Nullspace_maps/2(A), grad w/1(A), Nullspace derivatives/2(A), Potential Function/1(A), Potential Function3/5(A)

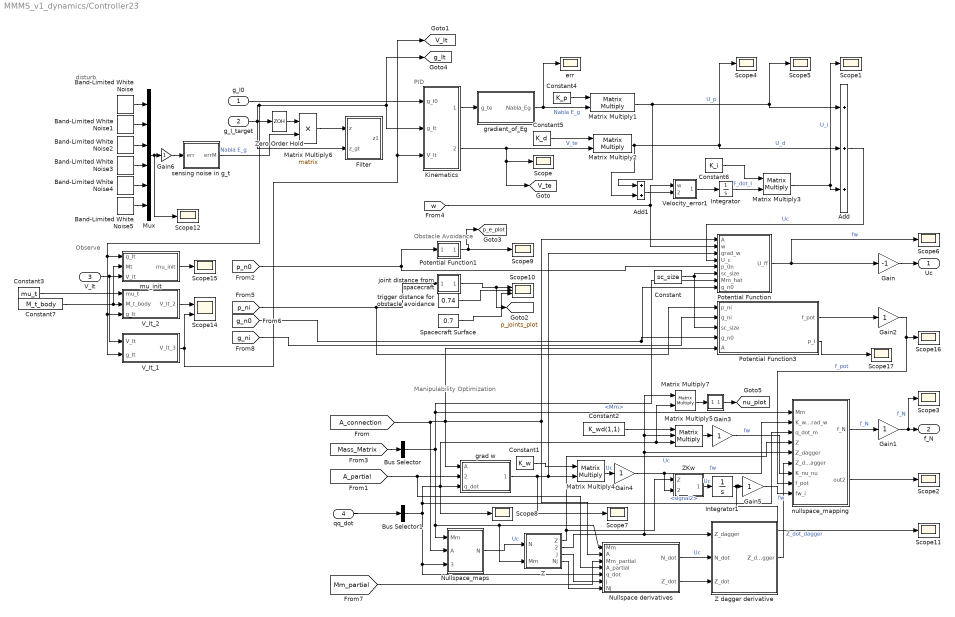
== system MMMS_v1_dynamics/Controller23 ==
  note: PID
  note: Manipulability Optimization
  note: Obstacle Avoidance
  note: Observe
  note: disturb
  g_I0 : Inport
  g_I_target : Inport  Port=2
  V_It : Inport  Port=3
  qq_dot : Inport  Port=4
  " " : MATLAB Function  TreatAsAtomicUnit=on
  Add : Sum  Inputs=+++
  Add1 : Sum
  Band-Limited White Noise : simulink/Sources/Band-Limited White Noise  Cov=[0.000001]  Ts=0.1  seed=[23341]
  Band-Limited White Noise1 : simulink/Sources/Band-Limited White Noise  Cov=[0.000001]  Ts=0.1  seed=[23342]
  Band-Limited White Noise2 : simulink/Sources/Band-Limited White Noise  Cov=[0.000001]  Ts=0.1  seed=[23343]
  Band-Limited White Noise3 : simulink/Sources/Band-Limited White Noise  Cov=[0.000001]  Ts=0.1  seed=[23344]
  Band-Limited White Noise4 : simulink/Sources/Band-Limited White Noise  Cov=[0.000001]  Ts=0.1  seed=[23345]
  Band-Limited White Noise5 : simulink/Sources/Band-Limited White Noise  Cov=[0.000001]  Ts=0.1  seed=[23346]
  Bus Selector : BusSelector  OutputSignals=Mm
  Bus Selector1 : BusSelector  OutputSignals=signal2
  Constant : Constant  Value=sc_size
  Constant1 : Constant  Value=K_w
  Constant2 : Constant  Value=K_wd(1,1)
  Constant3 : Constant  Value=mu_t
  Constant4 : Constant  Value=K_p
  Constant5 : Constant  Value=K_d
  Constant6 : Constant  Value=K_i
  Constant7 : Constant  Value=M_t_body
  Filter : Subsystem
  Gain : Gain  Gain=-1
  Gain{1..6} (6 alike) : Gain
  Integrator : Integrator
  Integrator1 : Integrator
  Kinematics : Subsystem
  Matrix Multiply{1..4,6..7} (6 alike) : Product  Multiplication=Matrix(*)
  Matrix Multiply5 : Product  Inputs=3  Multiplication=Matrix(*)
  Mux : Mux  Inputs=6
  Nullspace derivatives : MATLAB Function  TreatAsAtomicUnit=on
  Nullspace_maps : MATLAB Function  TreatAsAtomicUnit=on
  Potential Function : MATLAB Function  TreatAsAtomicUnit=on
  Potential Function1 : MATLAB Function  TreatAsAtomicUnit=on
  Potential Function3 : MATLAB Function  TreatAsAtomicUnit=on
  Scope{,1..9,11..12,15..17} (15 alike) : Scope
  Scope10 : Scope  NumInputPorts=3
  Scope14 : Scope  NumInputPorts=2
  Spacecraft Surface : Constant  Value=0.7
  V_It_1 : MATLAB Function  TreatAsAtomicUnit=on
  V_It_2 : MATLAB Function  TreatAsAtomicUnit=on
  Velocity_error1 : MATLAB Function  TreatAsAtomicUnit=on
  Z : MATLAB Function  TreatAsAtomicUnit=on
  Z dagger derivative : MATLAB Function  TreatAsAtomicUnit=on
  ZKw : MATLAB Function  TreatAsAtomicUnit=on
  Zero-Order Hold : ZeroOrderHold  SampleTime=0.1
  err : Scope
  grad w : MATLAB Function  TreatAsAtomicUnit=on
  gradient_of_Eg : MATLAB Function  TreatAsAtomicUnit=on
  joint distance from spacecraft : MATLAB Function  TreatAsAtomicUnit=on
  mu_init : MATLAB Function  TreatAsAtomicUnit=on
  nullspace_mapping : MATLAB Function  TreatAsAtomicUnit=on
  sensing noise in g_t : MATLAB Function  TreatAsAtomicUnit=on
  trigger distance for obstacle avoidance : Constant  Value=0.74
  Uc : Outport
  f_N : Outport  Port=2
  tag scope: V_It=global, V_te=global, g_It=global, nu_plot=global, p_e_plot=global, p_joints_plot=global
  wires:
  [A_connection] -> Potential Function3/5(A), Potential Function/1(A), Nullspace derivatives/2(A), grad w/1(A), Nullspace_maps/2(A)
  [A_partial] -> grad w/2(A_partial), Nullspace derivatives/4(A_partial)
  qq_dot/1 -> Bus Selector1/1
  [Mass_Matrix] -> Bus Selector/1
  Bus Selector/1 -> Nullspace_maps/1(Mm), Z/2(Mm), Nullspace derivatives/1(Mm), Potential Function/7(Mm_hat), nullspace_mapping/1(Mm)  "<Mm>"
  Gain/1 -> Uc/1
  g_I0/1 -> Kinematics/1(g_I0)
  Add/1 -> Potential Function/4(U_c)  "Uc"
  Kinematics/1(g_te1) -> gradient_of_Eg/1(g_te)
  Add1/1 -> Velocity_error1/2(in)
  Matrix Multiply2/1 -> Scope4/1, Add/2, Add1/2  "U_d"
  gradient_of_Eg/1(Nabla_Eg) -> err/1, Matrix Multiply1/2  "Nabla E_g"
  Constant4/1 -> Matrix Multiply1/1
  Kinematics/2(V_te) -> [V_te], Scope/1, Matrix Multiply2/2  "V_te"
  Constant6/1 -> Matrix Multiply3/1
  Integrator/1 -> Matrix Multiply3/2  "F_dot_I"
  Matrix Multiply1/1 -> Scope5/1, Add/1, Add1/1  "U_p"
  Constant5/1 -> Matrix Multiply2/1
  Bus Selector1/1 -> nullspace_mapping/3(q_dot_m), Scope8/1, grad w/3(q_dot), Matrix Multiply7/2, Matrix Multiply5/3, Nullspace derivatives/5(q_dot), Nullspace_maps/3(q_dot_m)  "<signal2>"
  Gain1/1 -> f_N/1, Scope3/1  "f_N"
  Constant1/1 -> Matrix Multiply4/1
  grad w/1(grad_w) -> Scope7/1, Potential Function/3(grad_w), Matrix Multiply4/2
  Matrix Multiply5/1 -> Gain3/1
  Constant2/1 -> Matrix Multiply5/1
  Matrix Multiply4/1 -> Gain4/1  "Uc"
  Matrix Multiply3/1 -> Scope1/1, Add/3  "U_i"
  nullspace_mapping/1(f_N) -> Gain1/1  "f_N"
  [w] -> Potential Function/2(w), Velocity_error1/1(w)
  Potential Function/1(U_ff) -> Scope6/1, Gain/1  "fw"
  Velocity_error1/1(out) -> Integrator/1
  [p_n0] -> Potential Function1/1(p_0n), Potential Function/5(p_0n)
  Potential Function1/1(w_p) -> Scope9/1, [p_e_plot]
  [p_ni] -> joint distance from spacecraft/1(p_joints), Potential Function3/1(p_ni)
  joint distance from spacecraft/1(pnorm) -> [p_joints_plot], Scope10/1
  [g_n0] -> Potential Function3/4(g_n0), Potential Function/8(g_n0)
  Potential Function3/1(f_pot) -> Gain2/1
  Constant/1 -> Potential Function3/3(sc_size), Potential Function/6(sc_size)
  trigger distance for obstacle avoidance/1 -> Scope10/2
  Gain3/1 -> nullspace_mapping/7(K_nu_nu)  "fw"
  Nullspace derivatives/1(N_dot) -> Z dagger derivative/2(N_dot)  "Uc"
  Nullspace derivatives/2(Z_dot) -> Z dagger derivative/3(Z_dot)
  Z dagger derivative/1(Z_dot_dagger) -> nullspace_mapping/6(Z_dot_dagger)  "Z_dot_dagger"
  Nullspace_maps/1(N) -> Z/1(N)  "Uc"
  [Mm_partial] -> Nullspace derivatives/3(Mm_partial)
  Z/1(Z) -> ZKw/1(Z), nullspace_mapping/4(Z)  "Uc"
  Gain4/1 -> ZKw/2(K_w_grad_w), nullspace_mapping/2(K_w_grad_w)  "fw"
  nullspace_mapping/2(out2) -> Scope2/1
  Z/2(Z_dagger) -> Z dagger derivative/1(Z_dagger), nullspace_mapping/5(Z_dagger), Matrix Multiply7/1, Matrix Multiply5/2
  ZKw/1(out) -> Integrator1/1  "Uc"
  Integrator1/1 -> Scope11/1, Gain5/1
  Gain5/1 -> nullspace_mapping/9(fw_i)  "fw"
  V_It/1 -> V_It_1/1(V_It), mu_init/3(V_It)
  Constant3/1 -> V_It_2/1(mu_t)
  mu_init/1(mu_init) -> Scope15/1
  Constant7/1 -> mu_init/2(Mt), V_It_2/2(M_t_body)
  Gain2/1 -> Scope16/1, nullspace_mapping/8(f_pot)  "f_pot"
  Band-Limited White Noise/1 -> Mux/1
  sensing noise in g_t/1(errM) -> Matrix Multiply6/2  "Nabla E_g"
  Mux/1 -> Scope12/1, Gain6/1
  Band-Limited White Noise2/1 -> Mux/3
  Band-Limited White Noise4/1 -> Mux/5
  Band-Limited White Noise3/1 -> Mux/4
  Band-Limited White Noise5/1 -> Mux/6
  Band-Limited White Noise1/1 -> Mux/2
  Zero-Order Hold/1 -> Matrix Multiply6/1
  Z/3(j) -> Nullspace derivatives/6(j)
  Z/4(Nj) -> Nullspace derivatives/7(Nj)
  Gain6/1 -> sensing noise in g_t/1(err)
  V_It_2/1(V_It_2) -> Scope14/1
  V_It_1/1(V_It_3) -> Scope14/2, Kinematics/3(V_It), [V_It]
  Spacecraft Surface/1 -> Scope10/3
  [g_ni] -> Potential Function3/2(g_ni)
  Potential Function3/2(p_i) -> Scope17/1
  g_I_target/1 -> V_It_1/2(g_It), V_It_2/3(g_It), mu_init/1(g_It), Kinematics/2(g_It), [g_It], Filter/2(z_gt), Zero-Order Hold/1
  Matrix Multiply6/1 -> Filter/1(z)
  " "/1(normA) -> [nu_plot]
  Matrix Multiply7/1 -> " "/1(A)

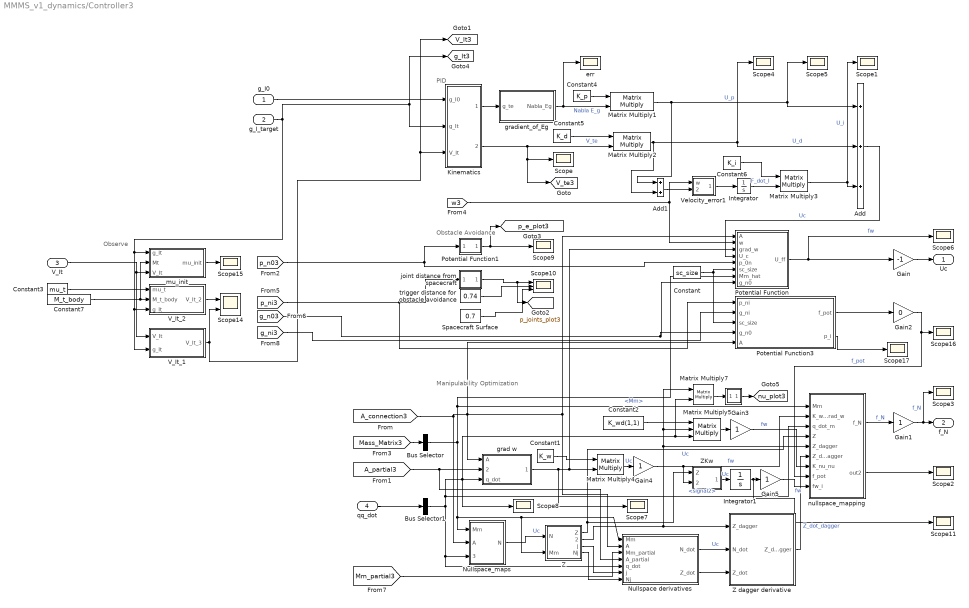
== system MMMS_v1_dynamics/Controller3 ==
  note: PID
  note: Manipulability Optimization
  note: Obstacle Avoidance
  note: Observe
  g_I0 : Inport
  g_I_target : Inport  Port=2
  V_It : Inport  Port=3
  qq_dot : Inport  Port=4
  " " : MATLAB Function  TreatAsAtomicUnit=on
  Add : Sum  Inputs=+++
  Add1 : Sum
  Bus Selector : BusSelector  OutputSignals=Mm
  Bus Selector1 : BusSelector  OutputSignals=signal2
  Constant : Constant  Value=sc_size
  Constant1 : Constant  Value=K_w
  Constant2 : Constant  Value=K_wd(1,1)
  Constant3 : Constant  Value=mu_t
  Constant4 : Constant  Value=K_p
  Constant5 : Constant  Value=K_d
  Constant6 : Constant  Value=K_i
  Constant7 : Constant  Value=M_t_body
  Gain : Gain  Gain=-1
  Gain{1,3..5} (4 alike) : Gain
  Gain2 : Gain  Gain=0
  Integrator : Integrator
  Integrator1 : Integrator
  Kinematics : Subsystem
  Matrix Multiply{1..4,7} (5 alike) : Product  Multiplication=Matrix(*)
  Matrix Multiply5 : Product  Inputs=3  Multiplication=Matrix(*)
  Nullspace derivatives : MATLAB Function  TreatAsAtomicUnit=on
  Nullspace_maps : MATLAB Function  TreatAsAtomicUnit=on
  Potential Function : MATLAB Function  TreatAsAtomicUnit=on
  Potential Function1 : MATLAB Function  TreatAsAtomicUnit=on
  Potential Function3 : MATLAB Function  TreatAsAtomicUnit=on
  Scope{,1..9,11,15..17} (14 alike) : Scope
  Scope10 : Scope  NumInputPorts=3
  Scope14 : Scope  NumInputPorts=2
  Spacecraft Surface : Constant  Value=0.7
  V_It_1 : MATLAB Function  TreatAsAtomicUnit=on
  V_It_2 : MATLAB Function  TreatAsAtomicUnit=on
  Velocity_error1 : MATLAB Function  TreatAsAtomicUnit=on
  Z : MATLAB Function  TreatAsAtomicUnit=on
  Z dagger derivative : MATLAB Function  TreatAsAtomicUnit=on
  ZKw : MATLAB Function  TreatAsAtomicUnit=on
  err : Scope
  grad w : MATLAB Function  TreatAsAtomicUnit=on
  gradient_of_Eg : MATLAB Function  TreatAsAtomicUnit=on
  joint distance from spacecraft : MATLAB Function  TreatAsAtomicUnit=on
  mu_init : MATLAB Function  TreatAsAtomicUnit=on
  nullspace_mapping : MATLAB Function  TreatAsAtomicUnit=on
  trigger distance for obstacle avoidance : Constant  Value=0.74
  Uc : Outport
  f_N : Outport  Port=2
  tag scope: V_It3=global, V_te3=global, g_It3=global, nu_plot3=global, p_e_plot3=global, p_joints_plot3=global
  wires:
  [A_connection3] -> Potential Function3/5(A), Potential Function/1(A), Nullspace derivatives/2(A), grad w/1(A), Nullspace_maps/2(A)
  [A_partial3] -> grad w/2(A_partial), Nullspace derivatives/4(A_partial)
  qq_dot/1 -> Bus Selector1/1
  [Mass_Matrix3] -> Bus Selector/1
  Bus Selector/1 -> Nullspace_maps/1(Mm), Z/2(Mm), Nullspace derivatives/1(Mm), Potential Function/7(Mm_hat), nullspace_mapping/1(Mm)  "<Mm>"
  Gain/1 -> Uc/1
  g_I0/1 -> Kinematics/1(g_I0)
  Add/1 -> Potential Function/4(U_c)  "Uc"
  Kinematics/1(g_te1) -> gradient_of_Eg/1(g_te)
  Add1/1 -> Velocity_error1/2(in)
  Matrix Multiply2/1 -> Scope4/1, Add/2, Add1/2  "U_d"
  gradient_of_Eg/1(Nabla_Eg) -> err/1, Matrix Multiply1/2  "Nabla E_g"
  Constant4/1 -> Matrix Multiply1/1
  Kinematics/2(V_te) -> [V_te3], Scope/1, Matrix Multiply2/2  "V_te"
  Constant6/1 -> Matrix Multiply3/1
  Integrator/1 -> Matrix Multiply3/2  "F_dot_I"
  Matrix Multiply1/1 -> Scope5/1, Add/1, Add1/1  "U_p"
  Constant5/1 -> Matrix Multiply2/1
  Bus Selector1/1 -> nullspace_mapping/3(q_dot_m), Scope8/1, grad w/3(q_dot), Matrix Multiply7/2, Matrix Multiply5/3, Nullspace derivatives/5(q_dot), Nullspace_maps/3(q_dot_m)  "<signal2>"
  Gain1/1 -> f_N/1, Scope3/1  "f_N"
  Constant1/1 -> Matrix Multiply4/1
  grad w/1(grad_w) -> Scope7/1, Potential Function/3(grad_w), Matrix Multiply4/2
  Matrix Multiply5/1 -> Gain3/1
  Constant2/1 -> Matrix Multiply5/1
  Matrix Multiply4/1 -> Gain4/1  "Uc"
  Matrix Multiply3/1 -> Scope1/1, Add/3  "U_i"
  nullspace_mapping/1(f_N) -> Gain1/1  "f_N"
  [w3] -> Potential Function/2(w), Velocity_error1/1(w)
  Potential Function/1(U_ff) -> Gain/1, Scope6/1  "fw"
  Velocity_error1/1(out) -> Integrator/1
  [p_n03] -> Potential Function1/1(p_0n), Potential Function/5(p_0n)
  Potential Function1/1(w_p) -> Scope9/1, [p_e_plot3]
  [p_ni3] -> joint distance from spacecraft/1(p_joints), Potential Function3/1(p_ni)
  joint distance from spacecraft/1(pnorm) -> [p_joints_plot3], Scope10/1
  [g_n03] -> Potential Function3/4(g_n0), Potential Function/8(g_n0)
  Potential Function3/1(f_pot) -> Gain2/1
  Constant/1 -> Potential Function3/3(sc_size), Potential Function/6(sc_size)
  trigger distance for obstacle avoidance/1 -> Scope10/2
  Gain3/1 -> nullspace_mapping/7(K_nu_nu)  "fw"
  Nullspace derivatives/1(N_dot) -> Z dagger derivative/2(N_dot)  "Uc"
  Nullspace derivatives/2(Z_dot) -> Z dagger derivative/3(Z_dot)
  Z dagger derivative/1(Z_dot_dagger) -> nullspace_mapping/6(Z_dot_dagger)  "Z_dot_dagger"
  Nullspace_maps/1(N) -> Z/1(N)  "Uc"
  [Mm_partial3] -> Nullspace derivatives/3(Mm_partial)
  Z/1(Z) -> ZKw/1(Z), nullspace_mapping/4(Z)  "Uc"
  Gain4/1 -> ZKw/2(K_w_grad_w), nullspace_mapping/2(K_w_grad_w)  "fw"
  nullspace_mapping/2(out2) -> Scope2/1
  Z/2(Z_dagger) -> Z dagger derivative/1(Z_dagger), nullspace_mapping/5(Z_dagger), Matrix Multiply7/1, Matrix Multiply5/2
  ZKw/1(out) -> Integrator1/1  "Uc"
  Integrator1/1 -> Scope11/1, Gain5/1
  Gain5/1 -> nullspace_mapping/9(fw_i)  "fw"
  V_It/1 -> V_It_1/1(V_It), mu_init/3(V_It)
  Constant3/1 -> V_It_2/1(mu_t)
  mu_init/1(mu_init) -> Scope15/1
  Constant7/1 -> mu_init/2(Mt), V_It_2/2(M_t_body)
  Gain2/1 -> Scope16/1, nullspace_mapping/8(f_pot)  "f_pot"
  Z/3(j) -> Nullspace derivatives/6(j)
  Z/4(Nj) -> Nullspace derivatives/7(Nj)
  V_It_2/1(V_It_2) -> Scope14/1
  V_It_1/1(V_It_3) -> Scope14/2, Kinematics/3(V_It), [V_It3]
  Spacecraft Surface/1 -> Scope10/3
  [g_ni3] -> Potential Function3/2(g_ni)
  Potential Function3/2(p_i) -> Scope17/1
  g_I_target/1 -> Kinematics/2(g_It), [g_It3], V_It_1/2(g_It), V_It_2/3(g_It), mu_init/1(g_It)
  " "/1(normA) -> [nu_plot3]
  Matrix Multiply7/1 -> " "/1(A)

== system MMMS_v1_dynamics/Dynamic Parameters ==
  note: Singularity of Jacobian
  note: Dynamic Parameters
  g_I0 : Inport
  q_ddot_m : Inport  Port=2
  " 1" : MATLAB Function  TreatAsAtomicUnit=on
  A_connection1 : Subsystem
  Bus Creator3 : BusCreator  Inputs=M0,M0m,Mm
  Bus Creator4 : BusCreator  Inputs=3
  Bus Selector : BusSelector  OutputSignals=signal1,signal2
  Constant1 : Constant  Value=mu
  Constant4 : Constant  Value=Xi_m
  Constant7 : Constant  Value=Xi_m_matrix
  MATLAB Function : MATLAB Function  TreatAsAtomicUnit=on
  MATLAB Function1 : MATLAB Function  TreatAsAtomicUnit=on
  Mass Matrix Blocks1 : Subsystem
  V_I1 : MATLAB Function  TreatAsAtomicUnit=on
  manipulability : Scope  NumInputPorts=2
  trigger : Constant  Value=0.003
  tag scope: A_connection=global, L=global, Mass_Matrix=global, P=global, V_Ie=global, w=global, w_plot=global
  wires:
  MATLAB Function1/1(P) -> V_I1/1(P), [P]
  Constant1/1 -> MATLAB Function1/2(mu)
  g_I0/1 -> MATLAB Function1/1(g_I0), V_I1/5(g_I0)
  A_connection1/1(A) -> [A_connection], V_I1/2(A_connection)
  Mass Matrix Blocks1/1(M0) -> A_connection1/1(M0), V_I1/4(M0), Bus Creator3/1  "M0"
  Mass Matrix Blocks1/3(Mm) -> Bus Creator3/3  "Mm"
  Bus Creator3/1 -> [Mass_Matrix]
  Bus Creator4/1 -> [L]
  q_ddot_m/1 -> Bus Selector/1
  " 1"/2(Lm0) -> Mass Matrix Blocks1/2(Lm0), Bus Creator4/2
  " 1"/1(L0) -> Bus Creator4/1
  Constant4/1 -> " 1"/2(Xi_m)
  " 1"/3(Lm) -> Bus Creator4/3, Mass Matrix Blocks1/1(Lm)
  Constant7/1 -> Mass Matrix Blocks1/3(Xi_m_matrix)
  Mass Matrix Blocks1/2(M0m) -> Bus Creator3/2, A_connection1/2(M0m)  "M0m"
  Bus Selector/2 -> V_I1/3(q_dot_m)  "<signal2>"
  Bus Selector/1 -> " 1"/1(q_m)  "<signal1>"
  MATLAB Function/1(wt) -> [w_plot], [w], manipulability/1  "manipulability measure"
  [A_connection] -> MATLAB Function/1(A)
  trigger/1 -> manipulability/2
  V_I1/1(V_I0) -> [V_Ie]

== system MMMS_v1_dynamics/Dynamic Parameters1 ==
  note: Dynamic Parameters
  note: Singularity of Jacobian
  g_I0 : Inport
  q_ddot_m : Inport  Port=2
  " 1" : MATLAB Function  TreatAsAtomicUnit=on
  A_connection1 : Subsystem
  Bus Creator3 : BusCreator  Inputs=M0,M0m,Mm
  Bus Creator4 : BusCreator  Inputs=3
  Bus Selector : BusSelector  OutputSignals=signal1,signal2
  Constant1 : Constant  Value=mu
  Constant4 : Constant  Value=Xi_m
  Constant7 : Constant  Value=Xi_m_matrix
  MATLAB Function : MATLAB Function  TreatAsAtomicUnit=on
  MATLAB Function1 : MATLAB Function  TreatAsAtomicUnit=on
  Mass Matrix Blocks1 : Subsystem
  V_I1 : MATLAB Function  TreatAsAtomicUnit=on
  manipulability : Scope  NumInputPorts=2
  trigger : Constant  Value=0.003
  tag scope: A_connection2=global, L2=global, Mass_Matrix2=global, P2=global, V_Ie2=global, w2=global, w_plot2=global
  wires:
  V_I1/1(V_I0) -> [V_Ie2]
  trigger/1 -> manipulability/2
  [A_connection2] -> MATLAB Function/1(A)
  MATLAB Function/1(wt) -> manipulability/1, [w2], [w_plot2]  "manipulability measure"
  Bus Selector/1 -> " 1"/1(q_m)  "<signal1>"
  Bus Selector/2 -> V_I1/3(q_dot_m)  "<signal2>"
  Mass Matrix Blocks1/2(M0m) -> A_connection1/2(M0m), Bus Creator3/2  "M0m"
  Constant7/1 -> Mass Matrix Blocks1/3(Xi_m_matrix)
  " 1"/3(Lm) -> Mass Matrix Blocks1/1(Lm), Bus Creator4/3
  Constant4/1 -> " 1"/2(Xi_m)
  " 1"/1(L0) -> Bus Creator4/1
  " 1"/2(Lm0) -> Bus Creator4/2, Mass Matrix Blocks1/2(Lm0)
  q_ddot_m/1 -> Bus Selector/1
  Bus Creator4/1 -> [L2]
  Bus Creator3/1 -> [Mass_Matrix2]
  Mass Matrix Blocks1/3(Mm) -> Bus Creator3/3  "Mm"
  Mass Matrix Blocks1/1(M0) -> Bus Creator3/1, V_I1/4(M0), A_connection1/1(M0)  "M0"
  A_connection1/1(A) -> V_I1/2(A_connection), [A_connection2]
  g_I0/1 -> V_I1/5(g_I0), MATLAB Function1/1(g_I0)
  Constant1/1 -> MATLAB Function1/2(mu)
  MATLAB Function1/1(P) -> [P2], V_I1/1(P)

== system MMMS_v1_dynamics/Dynamic Parameters2 ==
  note: Singularity of Jacobian
  note: Dynamic Parameters
  g_I0 : Inport
  q_ddot_m : Inport  Port=2
  " 1" : MATLAB Function  TreatAsAtomicUnit=on
  A_connection1 : Subsystem
  Bus Creator3 : BusCreator  Inputs=M0,M0m,Mm
  Bus Creator4 : BusCreator  Inputs=3
  Bus Selector : BusSelector  OutputSignals=signal1,signal2
  Constant1 : Constant  Value=mu
  Constant4 : Constant  Value=Xi_m
  Constant7 : Constant  Value=Xi_m_matrix
  MATLAB Function : MATLAB Function  TreatAsAtomicUnit=on
  MATLAB Function1 : MATLAB Function  TreatAsAtomicUnit=on
  Mass Matrix Blocks1 : Subsystem
  V_I1 : MATLAB Function  TreatAsAtomicUnit=on
  manipulability : Scope  NumInputPorts=2
  trigger : Constant  Value=0.003
  tag scope: A_connection3=global, L3=global, Mass_Matrix3=global, P3=global, V_Ie3=global, w3=global, w_plot3=global
  wires:
  MATLAB Function1/1(P) -> V_I1/1(P), [P3]
  Constant1/1 -> MATLAB Function1/2(mu)
  g_I0/1 -> MATLAB Function1/1(g_I0), V_I1/5(g_I0)
  A_connection1/1(A) -> [A_connection3], V_I1/2(A_connection)
  Mass Matrix Blocks1/1(M0) -> A_connection1/1(M0), V_I1/4(M0), Bus Creator3/1  "M0"
  Mass Matrix Blocks1/3(Mm) -> Bus Creator3/3  "Mm"
  Bus Creator3/1 -> [Mass_Matrix3]
  Bus Creator4/1 -> [L3]
  q_ddot_m/1 -> Bus Selector/1
  " 1"/2(Lm0) -> Mass Matrix Blocks1/2(Lm0), Bus Creator4/2
  " 1"/1(L0) -> Bus Creator4/1
  Constant4/1 -> " 1"/2(Xi_m)
  " 1"/3(Lm) -> Bus Creator4/3, Mass Matrix Blocks1/1(Lm)
  Constant7/1 -> Mass Matrix Blocks1/3(Xi_m_matrix)
  Mass Matrix Blocks1/2(M0m) -> Bus Creator3/2, A_connection1/2(M0m)  "M0m"
  Bus Selector/2 -> V_I1/3(q_dot_m)  "<signal2>"
  Bus Selector/1 -> " 1"/1(q_m)  "<signal1>"
  MATLAB Function/1(wt) -> [w_plot3], [w3], manipulability/1  "manipulability measure"
  [A_connection3] -> MATLAB Function/1(A)
  trigger/1 -> manipulability/2
  V_I1/1(V_I0) -> [V_Ie3]

== system MMMS_v1_dynamics/Feedback Transformation ==
  note: Feedback Transformation
  g_I0 : Inport
  q_m : Inport  Port=2
  U_c2 : Inport  Port=3
  In5 : Inport  Port=4
  Add1 : Sum  Inputs=++++++
  Bus Selector1 : BusSelector  OutputSignals=signal2
  Constant1 : Constant  Value=mu
  Constant4 : Constant  Value=mu_t
  Gain10 : Gain
  Gain5 : Gain  Gain=0
  Gain7 : Gain  Gain=0
  Gain8 : Gain
  Gain9 : Gain  Gain=0
  Inverse Dynamics1 : Subsystem
  Matrix Multiply{1..3,8} (4 alike) : Product  Multiplication=Matrix(*)
  f_m : Outport
  wires:
  Inverse Dynamics1/2(F_mu) -> Matrix Multiply3/1
  Gain7/1 -> Add1/2
  Matrix Multiply1/1 -> Gain7/1
  Gain10/1 -> Add1/6
  Inverse Dynamics1/1(F_U) -> Matrix Multiply2/1
  Constant1/1 -> Matrix Multiply3/2  "mu"
  U_c2/1 -> Matrix Multiply2/2
  Inverse Dynamics1/5(N) -> Gain5/1
  Matrix Multiply8/1 -> Gain8/1
  Matrix Multiply3/1 -> Gain9/1
  Gain5/1 -> Add1/1
  In5/1 -> Gain10/1
  Matrix Multiply2/1 -> Add1/3  "f_m"
  Bus Selector1/1 -> Matrix Multiply1/2  "<signal2>"
  Add1/1 -> f_m/1  "f_m"
  Constant4/1 -> Matrix Multiply8/2  "mu_t"
  Gain9/1 -> Add1/4
  Inverse Dynamics1/4(F_m) -> Matrix Multiply1/1
  Inverse Dynamics1/3(F_t) -> Matrix Multiply8/1
  Gain8/1 -> Add1/5
  g_I0/1 -> Inverse Dynamics1/1(g_I0)
  q_m/1 -> Bus Selector1/1, Inverse Dynamics1/2("q_m ")

== system MMMS_v1_dynamics/Feedback Transformation1 ==
  note: Feedback Transformation
  g_I0 : Inport
  q_m : Inport  Port=2
  U_c2 : Inport  Port=3
  f_N : Inport  Port=4
  Add1 : Sum  Inputs=++++++
  Bus Selector1 : BusSelector  OutputSignals=signal2
  Constant1 : Constant  Value=mu
  Constant4 : Constant  Value=mu_t
  Gain10 : Gain
  Gain5 : Gain  Gain=0
  Gain7 : Gain  Gain=0
  Gain8 : Gain
  Gain9 : Gain  Gain=0
  Inverse Dynamics1 : Subsystem
  Matrix Multiply{1..3,8} (4 alike) : Product  Multiplication=Matrix(*)
  f_m : Outport
  wires:
  q_m/1 -> Inverse Dynamics1/2("q_m "), Bus Selector1/1
  g_I0/1 -> Inverse Dynamics1/1(g_I0)
  Gain8/1 -> Add1/5
  Inverse Dynamics1/3(F_t) -> Matrix Multiply8/1
  Inverse Dynamics1/4(F_m) -> Matrix Multiply1/1
  Gain9/1 -> Add1/4
  Constant4/1 -> Matrix Multiply8/2  "mu_t"
  Add1/1 -> f_m/1  "f_m"
  Bus Selector1/1 -> Matrix Multiply1/2  "<signal2>"
  Matrix Multiply2/1 -> Add1/3  "f_m"
  f_N/1 -> Gain10/1
  Gain5/1 -> Add1/1
  Matrix Multiply3/1 -> Gain9/1
  Matrix Multiply8/1 -> Gain8/1
  Inverse Dynamics1/5(N) -> Gain5/1
  U_c2/1 -> Matrix Multiply2/2
  Constant1/1 -> Matrix Multiply3/2  "mu"
  Inverse Dynamics1/1(F_U) -> Matrix Multiply2/1
  Gain10/1 -> Add1/6
  Matrix Multiply1/1 -> Gain7/1
  Gain7/1 -> Add1/2
  Inverse Dynamics1/2(F_mu) -> Matrix Multiply3/1

== system MMMS_v1_dynamics/Feedback Transformation2 ==
  note: Feedback Transformation
  g_I0 : Inport
  q_m : Inport  Port=2
  U_c2 : Inport  Port=3
  f_N : Inport  Port=4
  Add1 : Sum  Inputs=++++++
  Bus Selector1 : BusSelector  OutputSignals=signal2
  Constant1 : Constant  Value=mu
  Constant4 : Constant  Value=mu_t
  Gain10 : Gain
  Gain5 : Gain  Gain=0
  Gain7 : Gain  Gain=0
  Gain8 : Gain
  Gain9 : Gain  Gain=0
  Inverse Dynamics1 : Subsystem
  Matrix Multiply{1..3,8} (4 alike) : Product  Multiplication=Matrix(*)
  f_m : Outport
  wires:
  Inverse Dynamics1/2(F_mu) -> Matrix Multiply3/1
  Gain7/1 -> Add1/2
  Matrix Multiply1/1 -> Gain7/1
  Gain10/1 -> Add1/6
  Inverse Dynamics1/1(F_U) -> Matrix Multiply2/1
  Constant1/1 -> Matrix Multiply3/2  "mu"
  U_c2/1 -> Matrix Multiply2/2
  Inverse Dynamics1/5(N) -> Gain5/1
  Matrix Multiply8/1 -> Gain8/1
  Matrix Multiply3/1 -> Gain9/1
  Gain5/1 -> Add1/1
  f_N/1 -> Gain10/1
  Matrix Multiply2/1 -> Add1/3  "f_m"
  Bus Selector1/1 -> Matrix Multiply1/2  "<signal2>"
  Add1/1 -> f_m/1  "f_m"
  Constant4/1 -> Matrix Multiply8/2  "mu_t"
  Gain9/1 -> Add1/4
  Inverse Dynamics1/4(F_m) -> Matrix Multiply1/1
  Inverse Dynamics1/3(F_t) -> Matrix Multiply8/1
  Gain8/1 -> Add1/5
  g_I0/1 -> Inverse Dynamics1/1(g_I0)
  q_m/1 -> Bus Selector1/1, Inverse Dynamics1/2("q_m ")

== system MMMS_v1_dynamics/Inverse Dynamics ==
  note: f_m
  g_I0 : Inport
  "q_m " : Inport  Port=2
  A_dot : MATLAB Function  TreatAsAtomicUnit=on
  Bus Selector : BusSelector  OutputSignals=M0,Mm
  Bus Selector2 : BusSelector  OutputSignals=signal1,signal2
  C_hat : Subsystem  Commented=on
  C_hat1 : Subsystem
  Inverse Dynamics : Subsystem
  M0_dot : MATLAB Function  TreatAsAtomicUnit=on
  N_hat : Subsystem  Commented=on
  N_hat1 : Subsystem
  Scope : Scope
  F_U : Outport
  F_mu : Outport  Port=2
  F_t : Outport  Port=3
  F_m : Outport  Port=4
  N : Outport  Port=5
  wires:
  [P] -> N_hat1/5(P)
  [Mass_Matrix] -> Bus Selector/1
  Bus Selector/1 -> N_hat1/6(M0), Inverse Dynamics/2(<M0>)  "<M0>"
  g_I0/1 -> N_hat1/1(g_I0), Inverse Dynamics/1(g_I0)
  Inverse Dynamics/1(F_U) -> F_U/1
  Inverse Dynamics/2(F_mu) -> F_mu/1
  Inverse Dynamics/3(F_t) -> F_t/1
  Inverse Dynamics/4(F_m) -> F_m/1
  Bus Selector/2 -> Inverse Dynamics/3(Mm)  "<Mm>"
  Bus Selector2/1 -> N_hat1/2(q_m), C_hat1/1(q_m)  "<signal1>"
  Bus Selector2/2 -> A_dot/2(q_m_dot), M0_dot/2(q_m_dot), N_hat1/3(q_dot_m), C_hat1/2(q_dot_m)  "<signal2>"
  C_hat1/1(M0_partial) -> M0_dot/1(M0_partial)
  C_hat1/2(Out1) -> A_dot/1(A_partial)
  C_hat1/3(C_hat1) -> Inverse Dynamics/6(C_hat)
  M0_dot/1(M0_dot) -> Inverse Dynamics/4(M0_dot)
  A_dot/1(A_dot) -> Inverse Dynamics/5(A_dot)
  "q_m "/1 -> Bus Selector2/1
  [A_connection] -> N_hat1/4(A)
  N_hat1/1(N_hat1) -> N/1, Scope/1
